simulink model "crane"  (Simulink 7.6)
settings: Solver=ode45  StartTime=0.0  StopTime=10.0  FixedStep=0.01  RelTol=1e-3
InitFcn:
  | initialize
undefined symbols (not defined in the file): xref
settings Model: Creator=pgoulart  LastModifiedBy=milan
settings DataIOCC: SaveOutput=off  DSMLogging=off  SaveTime=off  SignalLoggingName=craneLogger
settings DebuggingCC: UnderspecifiedInitializationDetection=Simplified  SolverPrmCheckMsg=none

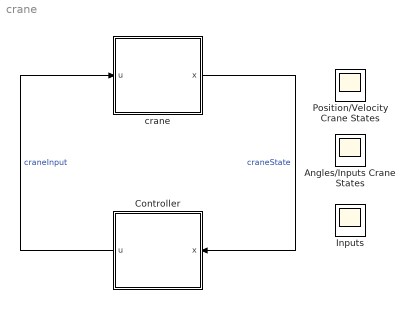
== system crane ==
  Angles/Inputs Crane States : Scope  NumInputPorts=4
      settings: Floating=on  TimeRange=10  YMin=-5~-5~-5~-5  YMax=5~5~5~5  SaveName=ScopeData2
  Controller : Subsystem
      mask init:
      | %initialize from data file
      | [data] = craneData;
      | 
      | %map to block-scoped variables
      | %-----------------------------
      | 
      | %constants
      | m       = data.simModel.m;
      | g       = data.simModel.g;
      | c       = data.simModel.c;
      | A_C     = data.simModel.A_C;
      | tau_C   = data.simModel.tau_C;
      | A_L     = data.simModel.A_L;
      | tau_L   = data.simModel.tau_L;
      | 
      | %initial states
      | x_C_init    = data.initialState.x_C;
      | x_L_init    = data.initialState.x_L;
      | v_C_init    = data.initialState.v_C;
      | v_L_init    = data.initialState.v_L;
      | theta_init  = data.initialState.theta;
      | omega_init  = data.initialState.omega;
      | u_C_init    = data.initialState.u_C;
      | u_L_init    = data.initialState.u_L;
      mask Display: disp('Controller');
  Inputs : Scope  NumInputPorts=2
      settings: Floating=on  TimeRange=10  YMin=-5~-5  YMax=5~5
  Position/Velocity Crane States : Scope  NumInputPorts=4
      settings: Floating=on  TimeRange=10  YMin=-5~-5~-5~-5  YMax=5~5~5~5
  crane : Subsystem
      mask help: KUL Lueven Crane Model. Edit <craneData.m> for configuration.
      mask init: same as crane/Controller
      mask Display: disp('Crane');
  wires:
  Controller/1(u) -> crane/1(u)  "craneInput"
  crane/1(x) -> Controller/1(x)  "craneState"

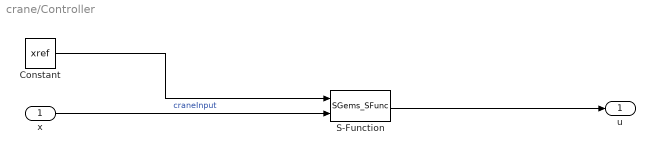
== system crane/Controller ==
  x : Inport
  Constant : Constant  Value=xref  OutDataTypeStr=Bus: xref_bus
  S-Function : S-Function  FunctionName=SGems_SFunc  EnableBusSupport=off
  u : Outport
  wires:
  S-Function/1 -> u/1
  Constant/1 -> S-Function/1
  x/1 -> S-Function/2  "craneInput"

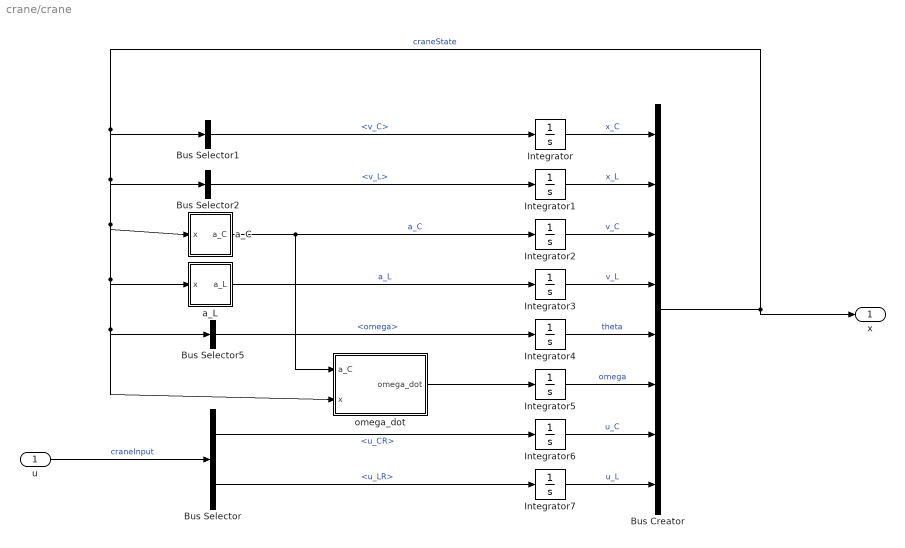
== system crane/crane ==
  u : Inport
  Bus Creator : BusCreator  Inputs='x_C','x_L','v_C','v_L','theta','omega','u_C','u_L'
  Bus Selector : BusSelector  OutputSignals=u_CR,u_LR
  Bus Selector1 : BusSelector  OutputSignals=v_C
  Bus Selector2 : BusSelector  OutputSignals=v_L
  Bus Selector5 : BusSelector  OutputSignals=omega
  Integrator : Integrator  InitialCondition=x_C_init
  Integrator1 : Integrator  InitialCondition=x_L_init
  Integrator2 : Integrator  InitialCondition=v_C_init
  Integrator3 : Integrator  InitialCondition=v_L_init
  Integrator4 : Integrator  InitialCondition=theta_init
  Integrator5 : Integrator  InitialCondition=omega_init
  Integrator6 : Integrator  InitialCondition=u_C_init
  Integrator7 : Integrator  InitialCondition=u_L_init
  a_C : Subsystem
  a_L : Subsystem
  omega_dot : Subsystem
  x : Outport
  wires:
  u/1 -> Bus Selector/1  "craneInput"
  Bus Selector1/1 -> Integrator/1  "<v_C>"
  Integrator/1 -> Bus Creator/1  "x_C"
  Integrator1/1 -> Bus Creator/2  "x_L"
  Integrator2/1 -> Bus Creator/3  "v_C"
  Integrator3/1 -> Bus Creator/4  "v_L"
  Integrator4/1 -> Bus Creator/5  "theta"
  Integrator5/1 -> Bus Creator/6  "omega"
  Integrator6/1 -> Bus Creator/7  "u_C"
  Integrator7/1 -> Bus Creator/8  "u_L"
  Bus Creator/1 -> Bus Selector1/1, Bus Selector2/1, a_C/1(x), Bus Selector5/1, omega_dot/2(x), a_L/1(x), x/1  "craneState"
  Bus Selector2/1 -> Integrator1/1  "<v_L>"
  Bus Selector5/1 -> Integrator4/1  "<omega>"
  Bus Selector/1 -> Integrator6/1  "<u_CR>"
  Bus Selector/2 -> Integrator7/1  "<u_LR>"
  a_C/1(a_C) -> Integrator2/1, omega_dot/1(a_C)  "a_C"
  a_L/1(a_L) -> Integrator3/1  "a_L"
  omega_dot/1(omega_dot) -> Integrator5/1

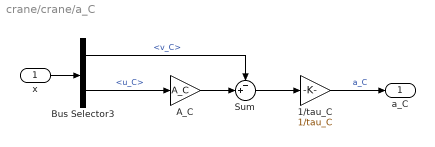
== system crane/crane/a_C ==
  x : Inport
  1/tau_C : Gain  Gain=1/tau_C
  A_C : Gain  Gain=A_C
  Bus Selector3 : BusSelector  OutputSignals=v_C,u_C
  Sum : Sum  Inputs=-+|
  a_C : Outport
  wires:
  1/tau_C/1 -> a_C/1  "a_C"
  x/1 -> Bus Selector3/1
  Bus Selector3/2 -> A_C/1  "<u_C>"
  A_C/1 -> Sum/2
  Sum/1 -> 1/tau_C/1
  Bus Selector3/1 -> Sum/1  "<v_C>"

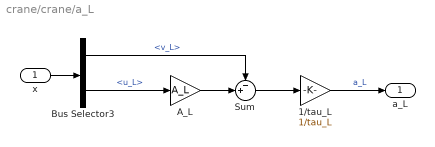
== system crane/crane/a_L ==
  x : Inport
  1/tau_L : Gain  Gain=1/tau_L
  A_L : Gain  Gain=A_L
  Bus Selector3 : BusSelector  OutputSignals=v_L,u_L
  Sum : Sum  Inputs=-+|
  a_L : Outport
  wires:
  1/tau_L/1 -> a_L/1  "a_L"
  x/1 -> Bus Selector3/1
  Bus Selector3/2 -> A_L/1  "<u_L>"
  A_L/1 -> Sum/2
  Sum/1 -> 1/tau_L/1
  Bus Selector3/1 -> Sum/1  "<v_L>"

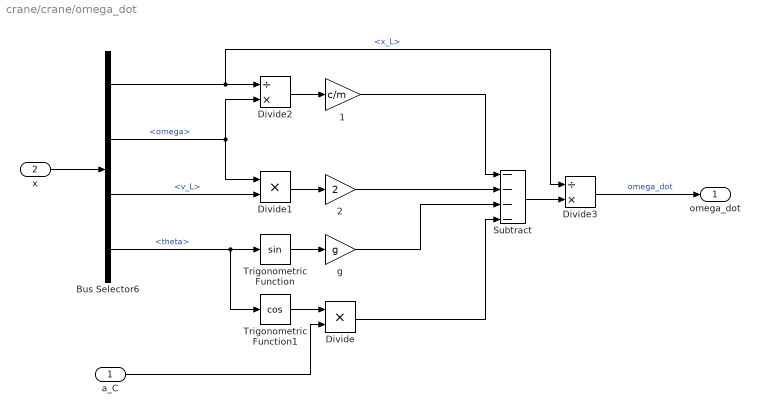
== system crane/crane/omega_dot ==
  a_C : Inport
  x : Inport  Port=2
  1 : Gain  Gain=c/m
  2 : Gain  Gain=2
  Bus Selector6 : BusSelector  OutputSignals=x_L,omega,v_L,theta
  Divide : Product  Inputs=**
  Divide1 : Product  Inputs=**
  Divide2 : Product  Inputs=/*
  Divide3 : Product  Inputs=/*
  Subtract : Sum  Inputs=----
  Trigonometric Function : Trigonometry
  Trigonometric Function1 : Trigonometry  Operator=cos
  g : Gain  Gain=g
  omega_dot : Outport
  wires:
  Trigonometric Function/1 -> g/1
  Divide1/1 -> 2/1
  Bus Selector6/2 -> Divide1/1, Divide2/2  "<omega>"
  Bus Selector6/3 -> Divide1/2  "<v_L>"
  Bus Selector6/1 -> Divide2/1, Divide3/1  "<x_L>"
  Divide2/1 -> 1/1
  2/1 -> Subtract/2
  1/1 -> Subtract/1
  Subtract/1 -> Divide3/2
  Divide3/1 -> omega_dot/1  "omega_dot"
  x/1 -> Bus Selector6/1
  Trigonometric Function1/1 -> Divide/1
  a_C/1 -> Divide/2
  g/1 -> Subtract/3
  Divide/1 -> Subtract/4
  Bus Selector6/4 -> Trigonometric Function/1, Trigonometric Function1/1  "<theta>"
